simulink model "SCADA_Sawmill"  (R2024b)
settings: Solver=FixedStepAuto  StartTime=0.0  StopTime=Tsim  FixedStep=dT  RelTol=1e-3
values from neighbouring files (symbols this model uses):
  b = t + 2*s    (= 3.6)    [ParametriSegheria.m]    (also in ParametriSegheriaDinamica.m; main_param_CLASSIC.m; main_param_SCADA.m)
  change_cost = 60    [ParametriSegheriaDinamica.m]    (also in main_param_CLASSIC.m = 50; main_param_SCADA.m = 50)
  dT = 0.025    [ParametriSegheriaDinamica.m]    (also in main_param_CLASSIC.m; main_param_SCADA.m)
  h_index = [70, 80, 90, 100]    [ParametriSegheria.m]    (also in ParametriSegheriaDinamica.m = [80, 90, 100]; main_param_CLASSIC.m = [80, 90, 100, 110]; main_param_SCADA.m = [80, 90, 100, 110])
  h_start_1 = 1    [main_param_CLASSIC.m]
  h_start_2 = 2    [main_param_CLASSIC.m]
  h_start_3 = 3    [main_param_CLASSIC.m]
  h_start_4 = 1    [main_param_CLASSIC.m]
  h_start_5 = 2    [main_param_CLASSIC.m]
  h_start_6 = 3    [main_param_CLASSIC.m]
  J1 = 8*1e6    (= 8000000)    [ParametriSegheriaDinamica.m]    (also in main_param_CLASSIC.m; main_param_SCADA.m)
  J2 = 0.9*1e6    (= 900000)    [ParametriSegheriaDinamica.m]    (also in main_param_CLASSIC.m; main_param_SCADA.m)
  kc = [0 35 40 50 55 90]    [ParametriSegheria.m]    (also in ParametriSegheriaDinamica.m = [0, 25, 30, 35, 50, 70]; main_param_CLASSIC.m = [0, 25, 30, 35, 50, 70]; main_param_SCADA.m = [0, 25, 30, 35, 50, 70])
  Kt = 2    [ParametriSegheria.m]    (also in ParametriSegheriaDinamica.m = 10000; main_param_CLASSIC.m = 10000; main_param_SCADA.m = 10000)
  Kt2 = 5    [ParametriSegheria.m]    (also in ParametriSegheriaDinamica.m = 4500; main_param_CLASSIC.m = 4500; main_param_SCADA.m = 4500)
  l_index = [20, 30, 40, 50]    [ParametriSegheria.m]    (also in ParametriSegheriaDinamica.m = [30, 40, 50]; main_param_CLASSIC.m = [30, 40, 50, 60]; main_param_SCADA.m = [30, 40, 50, 60])
  l_start_1 = 1    [main_param_CLASSIC.m]
  l_start_2 = 1    [main_param_CLASSIC.m]
  l_start_3 = 1    [main_param_CLASSIC.m]
  l_start_4 = 1    [main_param_CLASSIC.m]
  l_start_5 = 1    [main_param_CLASSIC.m]
  l_start_6 = 1    [main_param_CLASSIC.m]
  Lt = 4    [ParametriSegheria.m]    (also in ParametriSegheriaDinamica.m; main_param_CLASSIC.m; main_param_SCADA.m)
  Mag_D1 = [0 randi([220 500], 1, 40)]    [ParametriSegheria.m]    (also in ParametriSegheriaDinamica.m = [0 randi([200 500], 1, N_log)]; main_param_CLASSIC.m = [0 randi([200 500], 1, N_log)]; main_param_SCADA.m = [0 randi([200 500], 1, N_log)])
  Mag_D2 = [0 randi([220 500], 1, 40)]    [ParametriSegheria.m]    (also in ParametriSegheriaDinamica.m = [0 randi([200 500], 1, N_log)]; main_param_CLASSIC.m = [0 randi([200 500], 1, N_log)]; main_param_SCADA.m = [0 randi([200 500], 1, N_log)])
  Mag_D3 = [0 randi([220 500], 1, 40)]    [ParametriSegheria.m]    (also in ParametriSegheriaDinamica.m = [0 randi([200 500], 1, N_log)]; main_param_CLASSIC.m = [0 randi([200 500], 1, N_log)]; main_param_SCADA.m = [0 randi([200 500], 1, N_log)])
  Mag_legno1 = [0 randi([1 5], 1, 40)]    [ParametriSegheria.m]    (also in ParametriSegheriaDinamica.m = [0 randi([1 5], 1, N_log)]; main_param_CLASSIC.m = [0 randi([1 5], 1, N_log)]; main_param_SCADA.m = [0 randi([1 5], 1, N_log)])
  Mag_legno2 = [0 randi([1 5], 1, 40)]    [ParametriSegheria.m]    (also in ParametriSegheriaDinamica.m = [0 randi([1 5], 1, N_log)]; main_param_CLASSIC.m = [0 randi([1 5], 1, N_log)]; main_param_SCADA.m = [0 randi([1 5], 1, N_log)])
  Mag_legno3 = [0 randi([1 5], 1, 40)]    [ParametriSegheria.m]    (also in ParametriSegheriaDinamica.m = [0 randi([1 5], 1, N_log)]; main_param_CLASSIC.m = [0 randi([1 5], 1, N_log)]; main_param_SCADA.m = [0 randi([1 5], 1, N_log)])
  n_linee = 3    [ParametriSegheriaDinamica.m]    (also in main_param_CLASSIC.m; main_param_SCADA.m)
  omega_ref1 = 50    [ParametriSegheriaDinamica.m]    (also in main_param_CLASSIC.m; main_param_SCADA.m)
  omega_ref2 = 3000*(2*pi/60)    (= 314.159265359)    [ParametriSegheriaDinamica.m]    (also in main_param_CLASSIC.m; main_param_SCADA.m)
  Rc = 200    [ParametriSegheria.m]    (also in ParametriSegheriaDinamica.m; main_param_CLASSIC.m; main_param_SCADA.m)
  rho = [0, 450, 520, 590, 710, 780]*1e-9    [ParametriSegheriaDinamica.m]    (also in main_param_CLASSIC.m; main_param_SCADA.m)
  Rs = 800    [ParametriSegheria.m]    (also in ParametriSegheriaDinamica.m; main_param_CLASSIC.m; main_param_SCADA.m)
  sigma_D = 10    [ParametriSegheriaDinamica.m]    (also in main_param_CLASSIC.m = 5; main_param_SCADA.m = 5)
  sigma_larg = 10    [ParametriSegheriaDinamica.m]    (also in main_param_CLASSIC.m = 5; main_param_SCADA.m = 5)
  SR = Rs/Rm    (= 5.33333333333)    [ParametriSegheria.m]    (also in ParametriSegheriaDinamica.m; main_param_CLASSIC.m; main_param_SCADA.m)
  SR2 = Rc/Rm2    (= 4)    [ParametriSegheria.m]    (also in ParametriSegheriaDinamica.m; main_param_CLASSIC.m; main_param_SCADA.m)
  target_matrice = randi([20, 120], length(h_index), length(l_index))    [ParametriSegheria.m]    (also in ParametriSegheriaDinamica.m = randi([20, 100], length(h_index), length(l_index)); main_param_CLASSIC.m = randi([20, 100], length(h_index), length(l_index)); main_param_SCADA.m = randi([20, 100], length(h_index), length(l_index)))
  thr_lavoro = 600000    [ParametriSegheriaDinamica.m]    (also in main_param_CLASSIC.m; main_param_SCADA.m)
  V_mean1 = 0.75    [ParametriSegheriaDinamica.m]    (also in main_param_CLASSIC.m; main_param_SCADA.m)
  V_mean23 = 1    [ParametriSegheriaDinamica.m]    (also in main_param_CLASSIC.m; main_param_SCADA.m)
libraries: simulink x24, slpidlib x18
(part 1 of 5)
settings Model: Creator=samue  LastModifiedBy=eliasantuari
settings SolverCC: EnableFixedStepZeroCrossing=on

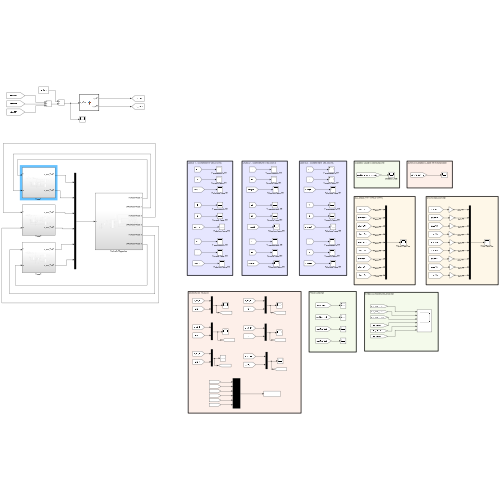
[thumbnail: Simulink's stored preview of the top-level diagram]
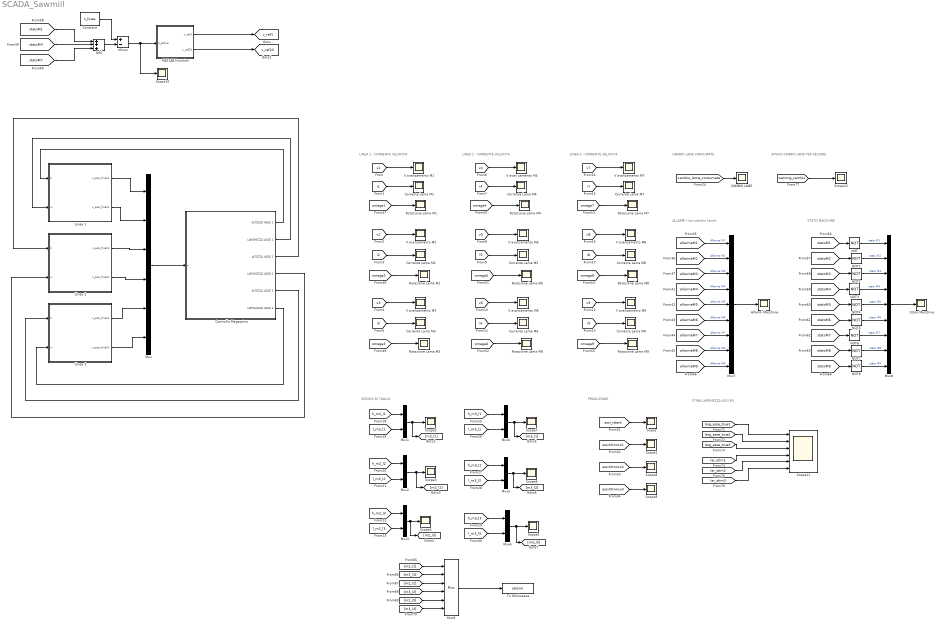
== system SCADA_Sawmill ==
  note: ALLARMI (non cambio lame)
  note: LINEA 2 - CORRENTE VELOCITA
  note: LINEA 1 - CORRENTE VELOCITA`
  note: LINEA 3 - CORRENTE VELOCITA
  note: SEZIONI DI TAGLIO
  note: CAMBIO LAME CONSUMATE
  note: PRODUZIONE
  note: STATO MACCHINE
  note: STIMA LARGHEZZA ASSI M1
  note: AVVISO CAMBIO LAME PER SEZIONE
  Add : Sum  Inputs=+++
  Allarmi Macchine : Scope
  CAMBIO LAME : Scope
  Constant : Constant  Value=n_linee
  Controllo Magazzino : Subsystem
  Corrente Lama M{1..9} (9 alike) : Scope
  Linea 1 : Subsystem
  Linea 2 : Subsystem
  Linea 3 : Subsystem
  MATLAB Function : MATLAB Function  TreatAsAtomicUnit=on
  Minus : Sum  Inputs=+-
  Mux : Mux  Inputs=6
  Mux{1..6} (6 alike) : Mux  Inputs=2
  Mux7 : Mux  Inputs=9
  Mux8 : Mux  Inputs=9
  Mux9 : Mux  Inputs=6
  NOT{,1..8} (9 alike) : Logic  Operator=NOT  IconShape=distinctive  AllPortsSameDT=off  OutDataTypeStr=boolean
  Rotazione Lama M{1..9} (9 alike) : Scope
  Scope{,1..10,12} (12 alike) : Scope
  Scope11 : Scope  NumInputPorts=6
  Stato Macchine : Scope
  To Workspace : ToWorkspace  VariableName=sezioni  SaveFormat=Timeseries  SampleTime=-1
  V avan zamento M4 : Scope
  V avanzamento M{1..3,5..9} (8 alike) : Scope
  tag scope: v_ref1=global, v_ref23=global
  wires:
  Linea 2/1(n_assi_finali1) -> Mux/3
  Controllo Magazzino/2(LARGHEZZA ASSE 1) -> Linea 1/2(w)
  Linea 2/2(n_assi_finali2) -> Mux/4
  [i9] -> Corrente Lama M9/1
  [v9] -> V avanzamento M9/1
  [i8] -> Corrente Lama M8/1
  [v7] -> V avanzamento M7/1
  [v8] -> V avanzamento M8/1
  [i7] -> Corrente Lama M7/1
  Controllo Magazzino/6(LARGHEZZA ASSE 3) -> Linea 3/2(w)
  Controllo Magazzino/3(ALTEZZA ASSE 2) -> Linea 2/1(h)
  [i3] -> Corrente Lama M3/1
  [v2] -> V avanzamento M2/1
  [v1] -> V avanzamento M1/1
  Controllo Magazzino/1(ALTEZZA ASSE 1) -> Linea 1/1(h)
  [i2] -> Corrente Lama M2/1
  [i1] -> Corrente Lama M1/1
  Linea 1/1(n_assi_finali1) -> Mux/1
  [v3] -> V avanzamento M3/1
  Mux/1 -> Controllo Magazzino/1(u)
  Linea 3/2(n_assi_finali2) -> Mux/6
  [i5] -> Corrente Lama M5/1
  [v5] -> V avanzamento M5/1
  Linea 3/1(n_assi_finali1) -> Mux/5
  Linea 1/2(n_assi_finali2) -> Mux/2
  [i4] -> Corrente Lama M4/1
  [v4] -> V avan zamento M4/1
  [v6] -> V avanzamento M6/1
  [i6] -> Corrente Lama M6/1
  Controllo Magazzino/5(ALTEZZA ASSE 3) -> Linea 3/1(h)
  Controllo Magazzino/4(LARGHEZZA ASSE 2) -> Linea 2/2(w)
  [cambio_lame_consumate] -> CAMBIO LAME/1
  [l_m2_l1] -> Mux1/2
  [h_m2_l1] -> Mux1/1
  Mux1/1 -> Scope2/1, [m2_l1]
  [h_m2_l2] -> Mux2/1
  [l_m2_l2] -> Mux2/2
  Mux2/1 -> [m2_l2], Scope3/1
  Mux3/1 -> Scope4/1, [m2_l3]
  [h_m2_l3] -> Mux3/1
  [l_m2_l3] -> Mux3/2
  Mux4/1 -> [m3_l3], Scope5/1
  [h_m3_l3] -> Mux4/1
  [l_m3_l3] -> Mux4/2
  Mux5/1 -> Scope6/1, [m3_l2]
  [h_m3_l2] -> Mux5/1
  [l_m3_l2] -> Mux5/2
  Mux6/1 -> [m3_l1], Scope7/1
  [h_m3_l1] -> Mux6/1
  [l_m3_l1] -> Mux6/2
  [assi_istant] -> Scope/1
  [assiXtronco1] -> Scope1/1
  [assiXtronco2] -> Scope8/1
  [assiXtronco3] -> Scope9/1
  [allarmeM3] -> Mux7/3  "Allarme M3"
  [allarmeM2] -> Mux7/2  "Allarme M2"
  Mux7/1 -> Allarmi Macchine/1
  [allarmeM1] -> Mux7/1  "Allarme M1"
  [allarmeM4] -> Mux7/4  "Allarme M4"
  [allarmeM5] -> Mux7/5  "Allarme M5"
  [allarmeM6] -> Mux7/6  "Allarme M6"
  [allarmeM9] -> Mux7/9  "Allarme M8"
  [allarmeM8] -> Mux7/8  "Allarme M4"
  [allarmeM7] -> Mux7/7  "Allarme M7"
  [statoM4] -> Add/2
  [statoM1] -> Add/1
  [statoM7] -> Add/3
  Add/1 -> Minus/2
  Constant/1 -> Minus/1
  Minus/1 -> Scope10/1, MATLAB Function/1(n_attive)
  MATLAB Function/1(v_ref1) -> [v_ref1]
  MATLAB Function/2(v_ref23) -> [v_ref23]
  [omega1] -> Rotazione Lama M1/1
  [omega2] -> Rotazione Lama M2/1
  [omega3] -> Rotazione Lama M3/1
  [omega4] -> Rotazione Lama M4/1
  [omega5] -> Rotazione Lama M5/1
  [omega6] -> Rotazione Lama M6/1
  [omega7] -> Rotazione Lama M7/1
  [omega8] -> Rotazione Lama M8/1
  [omega9] -> Rotazione Lama M9/1
  Mux8/1 -> Stato Macchine/1
  [statoM1] -> NOT/1
  NOT/1 -> Mux8/1  "stato M1"
  [statoM2] -> NOT1/1
  [statoM3] -> NOT2/1
  NOT1/1 -> Mux8/2  "stato M2"
  NOT2/1 -> Mux8/3  "stato M3"
  NOT5/1 -> Mux8/6  "stato M6"
  NOT4/1 -> Mux8/5  "stato M5"
  [statoM6] -> NOT5/1
  [statoM5] -> NOT4/1
  NOT3/1 -> Mux8/4  "stato M4"
  [statoM4] -> NOT3/1
  [statoM7] -> NOT6/1
  NOT6/1 -> Mux8/7  "stato M7"
  [statoM8] -> NOT7/1
  [statoM9] -> NOT8/1
  NOT7/1 -> Mux8/8  "stato M8"
  NOT8/1 -> Mux8/9  "stato M9"
  [m3_l1] -> Mux9/2
  Mux9/1 -> To Workspace/1
  [m2_l3] -> Mux9/5
  [m2_l2] -> Mux9/3
  [m3_l2] -> Mux9/4
  [m3_l3] -> Mux9/6
  [m2_l1] -> Mux9/1
  [larg_asse_true1] -> Scope11/1
  [larg_asse_true2] -> Scope11/2
  [larg_asse_true3] -> Scope11/3
  [lar_stim1] -> Scope11/4
  [lar_stim2] -> Scope11/5
  [lar_stim3] -> Scope11/6
  [warning_cambio] -> Scope12/1

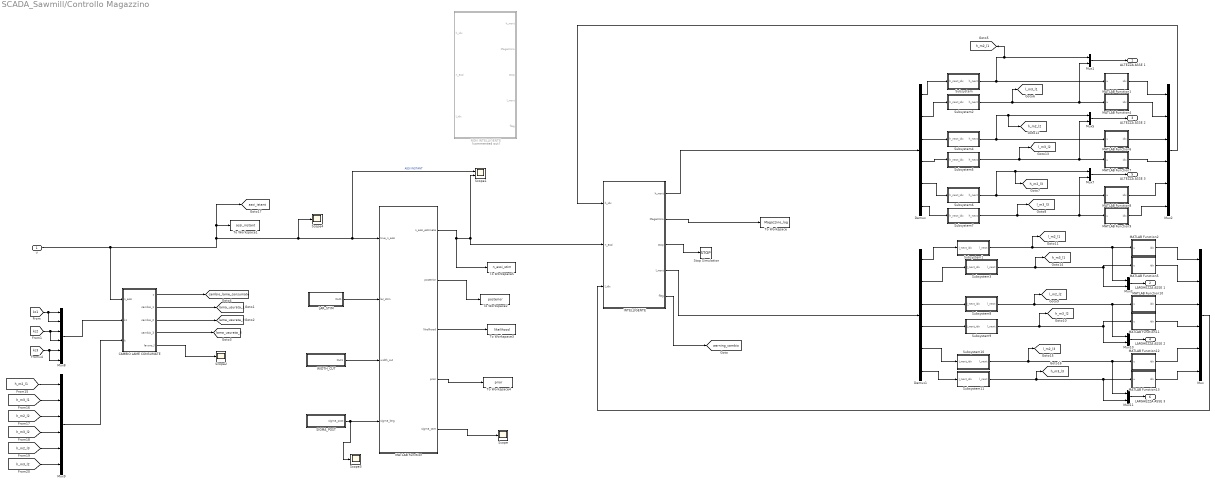
== system SCADA_Sawmill/Controllo Magazzino ==
  u : Inport
  CAMBIO LAME CONSUMATE : MATLAB Function  TreatAsAtomicUnit=on
  Demux : Demux  Outputs=6
  Demux1 : Demux  Outputs=6
  INTELLIGENTE : MATLAB Function  TreatAsAtomicUnit=on
  LAR_STIM : Subsystem
  MATLAB Function : MATLAB Function  TreatAsAtomicUnit=on
  MATLAB Function1 : MATLAB Function  TreatAsAtomicUnit=on
  MATLAB Function10 : MATLAB Function  TreatAsAtomicUnit=on
  MATLAB Function11 : MATLAB Function  TreatAsAtomicUnit=on
  MATLAB Function12 : MATLAB Function  TreatAsAtomicUnit=on
  MATLAB Function13 : MATLAB Function  TreatAsAtomicUnit=on
  MATLAB Function2 : MATLAB Function  TreatAsAtomicUnit=on
  MATLAB Function4 : MATLAB Function  TreatAsAtomicUnit=on
  MATLAB Function5 : MATLAB Function  TreatAsAtomicUnit=on
  MATLAB Function6 : MATLAB Function  TreatAsAtomicUnit=on
  MATLAB Function7 : MATLAB Function  TreatAsAtomicUnit=on
  MATLAB Function8 : MATLAB Function  TreatAsAtomicUnit=on
  MATLAB Function9 : MATLAB Function  TreatAsAtomicUnit=on
  Mux{,2,8..9} (4 alike) : Mux  Inputs=6
  Mux{1,3,5,7,10..11} (6 alike) : Mux  Inputs=2
  NON INTELLIGENTE : MATLAB Function  Commented=on  TreatAsAtomicUnit=on
  SIGMA_POST : Subsystem
  Scope{,2..4} (4 alike) : Scope
  Scope1 : Scope  NumInputPorts=2
  Stop Simulation : Stop
  Subsystem : Subsystem
  Subsystem1 : Subsystem
  Subsystem10 : Subsystem
  Subsystem11 : Subsystem
  Subsystem2 : Subsystem
  Subsystem3 : Subsystem
  Subsystem4 : Subsystem
  Subsystem5 : Subsystem
  Subsystem6 : Subsystem
  Subsystem7 : Subsystem
  Subsystem8 : Subsystem
  Subsystem9 : Subsystem
  To Workspace : ToWorkspace  VariableName=Magazzino_log  SaveFormat=Timeseries  SampleTime=-1
  To Workspace1 : ToWorkspace  VariableName=assi_instant  SaveFormat=Timeseries  SampleTime=-1
  To Workspace2 : ToWorkspace  VariableName=posterior  SaveFormat=Timeseries  SampleTime=-1
  To Workspace3 : ToWorkspace  VariableName=likelihood  SaveFormat=Timeseries  SampleTime=-1
  To Workspace4 : ToWorkspace  VariableName=prior  SaveFormat=Timeseries  SampleTime=-1
  To Workspace5 : ToWorkspace  VariableName=n_assi_stim  SaveFormat=Timeseries  SampleTime=-1
  WIDTH_CUT : Subsystem
  ALTEZZA ASSE 1 : Outport
  LARGHEZZA ASSE 1 : Outport  Port=2
  ALTEZZA ASSE 2 : Outport  Port=3
  LARGHEZZA ASSE 2 : Outport  Port=4
  ALTEZZA ASSE 3 : Outport  Port=5
  LARGHEZZA ASSE 3 : Outport  Port=6
  tag scope: assi_istant=global, cambio_lame_consumate=global, h_m2_l1=global, h_m2_l2=global, h_m2_l3=global, h_m3_l1=global, h_m3_l2=global, h_m3_l3=global, l_m2_l1=global, l_m2_l2=global, l_m2_l3=global, l_m3_l1=global, l_m3_l2=global, l_m3_l3=global, lama_usurata_1=global, lama_usurata_2=global, lama_usurata_3=global, warning_cambio=global
  wires:
  Subsystem/1(h_next) -> Mux1/1, [h_m2_l1], MATLAB Function1/1(u)
  Subsystem1/1(l_next) -> [l_m2_l1], Mux3/1, MATLAB Function2/1(u)
  Subsystem2/1(h_next) -> Mux1/2, MATLAB Function4/1(u), [l_m3_l1]
  Demux/2 -> Subsystem2/1(h_next_idx)
  Demux/1 -> Subsystem/1(h_next_idx)
  Mux1/1 -> ALTEZZA ASSE 1/1
  Subsystem3/1(l_next) -> [h_m3_l1], MATLAB Function5/1(u), Mux3/2
  Mux3/1 -> LARGHEZZA ASSE 1/1
  Subsystem5/1(h_next) -> [l_m3_l2], Mux5/2, MATLAB Function7/1(u)
  Mux5/1 -> ALTEZZA ASSE 2/1
  Subsystem4/1(h_next) -> [h_m2_l2], Mux5/1, MATLAB Function6/1(u)
  Subsystem7/1(h_next) -> [l_m3_l3], Mux7/2, MATLAB Function9/1(u)
  Mux7/1 -> ALTEZZA ASSE 3/1
  Subsystem6/1(h_next) -> [h_m2_l3], Mux7/1, MATLAB Function8/1(u)
  Demux/3 -> Subsystem4/1(h_next_idx)
  Demux/4 -> Subsystem5/1(h_next_idx)
  Demux/5 -> Subsystem6/1(h_next_idx)
  Demux/6 -> Subsystem7/1(h_next_idx)
  Mux10/1 -> LARGHEZZA ASSE 2/1
  Subsystem9/1(l_next) -> [h_m3_l2], MATLAB Function11/1(u), Mux10/2
  Subsystem8/1(l_next) -> [l_m2_l2], MATLAB Function10/1(u), Mux10/1
  Subsystem10/1(l_next) -> [l_m2_l3], Mux11/1, MATLAB Function12/1(u)
  Subsystem11/1(l_next) -> [h_m3_l3], Mux11/2, MATLAB Function13/1(u)
  Mux11/1 -> LARGHEZZA ASSE 3/1
  Demux1/1 -> Subsystem1/1(I_next_idx)
  Demux1/2 -> Subsystem3/1(I_next_idx)
  Demux1/3 -> Subsystem8/1(I_next_idx)
  Demux1/4 -> Subsystem9/1(I_next_idx)
  Demux1/5 -> Subsystem10/1(I_next_idx)
  Demux1/6 -> Subsystem11/1(I_next_idx)
  MATLAB Function2/1(idx) -> Mux/1
  MATLAB Function5/1(idx) -> Mux/2
  MATLAB Function10/1(idx) -> Mux/3
  MATLAB Function11/1(idx) -> Mux/4
  MATLAB Function12/1(idx) -> Mux/5
  MATLAB Function13/1(idx) -> Mux/6
  Mux/1 -> INTELLIGENTE/3(l_idx)
  MATLAB Function1/1(idx) -> Mux2/1
  MATLAB Function4/1(idx) -> Mux2/2
  MATLAB Function6/1(idx) -> Mux2/3
  MATLAB Function7/1(idx) -> Mux2/4
  MATLAB Function8/1(idx) -> Mux2/5
  MATLAB Function9/1(idx) -> Mux2/6
  Mux2/1 -> INTELLIGENTE/1(h_idx)
  INTELLIGENTE/2(Magazzino) -> To Workspace/1
  INTELLIGENTE/1(h_next) -> Demux/1
  INTELLIGENTE/4(l_next) -> Demux1/1
  INTELLIGENTE/3(stop) -> Stop Simulation/1
  MATLAB Function/2(posterior) -> To Workspace2/1
  MATLAB Function/3(likelihood) -> To Workspace3/1
  MATLAB Function/4(prior) -> To Workspace4/1
  [h_m3_l2] -> Mux9/6
  CAMBIO LAME CONSUMATE/3(cambio_2) -> [lama_usurata_2]
  [kc3] -> Mux8/6, Mux8/5
  u/1 -> CAMBIO LAME CONSUMATE/1(n_assi), Scope4/1, Scope1/1, MATLAB Function/1(true_n_assi), To Workspace1/1, [assi_istant]  "ASSI INSTANT"
  [kc1] -> Mux8/2, Mux8/1
  [kc2] -> Mux8/4, Mux8/3
  CAMBIO LAME CONSUMATE/4(cambio_3) -> [lama_usurata_3]
  CAMBIO LAME CONSUMATE/1(y) -> [cambio_lame_consumate]
  Mux8/1 -> CAMBIO LAME CONSUMATE/2(kc)
  [h_m2_l2] -> Mux9/3
  Mux9/1 -> CAMBIO LAME CONSUMATE/3(h)
  CAMBIO LAME CONSUMATE/5(lavoro_l) -> Scope2/1
  CAMBIO LAME CONSUMATE/2(cambio_1) -> [lama_usurata_1]
  [h_m3_l1] -> Mux9/2
  [h_m3_l2] -> Mux9/4
  [h_m2_l1] -> Mux9/1
  [h_m2_l3] -> Mux9/5
  WIDTH_CUT/1(Out1) -> MATLAB Function/3(width_cut)
  LAR_STIM/1(Out1) -> MATLAB Function/2(lar_stim)
  SIGMA_POST/1(sigma_post) -> Scope3/1, MATLAB Function/4(sigma_larg)
  MATLAB Function/1(n_assi_estimate) -> INTELLIGENTE/2(n_assi), Scope1/2, To Workspace5/1
  INTELLIGENTE/5(flag) -> [warning_cambio]
  MATLAB Function/5(sigma_cam) -> Scope/1

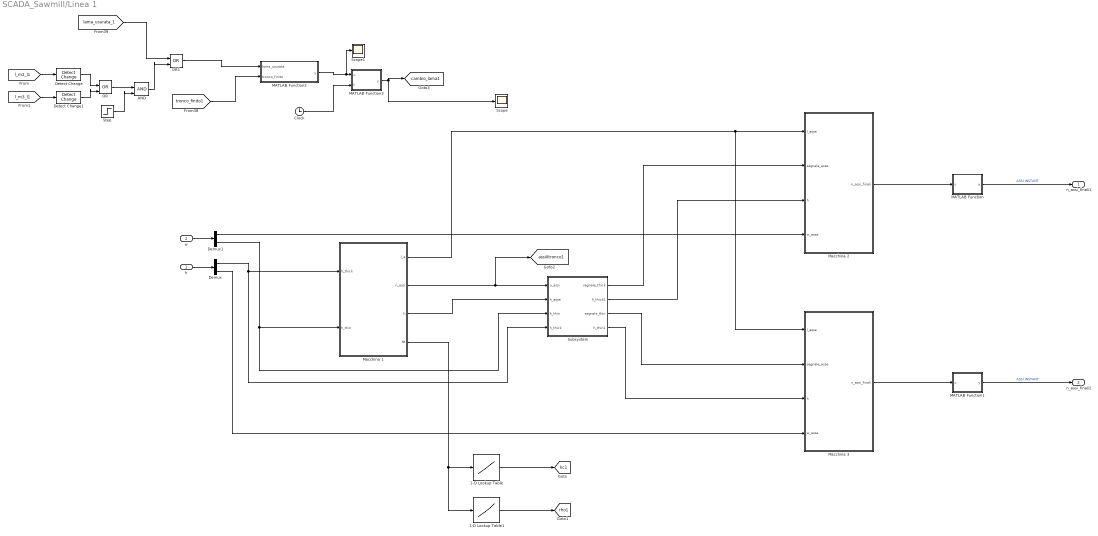
== system SCADA_Sawmill/Linea 1 ==
  h : Inport
  w : Inport  Port=2
  1-D Lookup Table : Lookup_n-D  NumberOfTableDimensions=1  BreakpointsForDimension1=[0 1 2 3 4 5 ]  Table=kc  InternalRulePriority=Speed  RndMeth=Simplest
  1-D Lookup Table1 : Lookup_n-D  NumberOfTableDimensions=1  BreakpointsForDimension1=[0 1 2 3 4 5 ]  Table=rho  InternalRulePriority=Speed  RndMeth=Simplest
  AND : Logic  IconShape=distinctive  AllPortsSameDT=off  OutDataTypeStr=boolean
  Clock : Clock
  Demux : Demux  Outputs=2
  Demux1 : Demux  Outputs=2
  Detect Change : simulink/Logic and Bit Operations/Detect Change  vinit=0  OutDataTypeStr=boolean
  Detect Change1 : simulink/Logic and Bit Operations/Detect Change  vinit=0  OutDataTypeStr=boolean
  MATLAB Function : MATLAB Function  TreatAsAtomicUnit=on
  MATLAB Function1 : MATLAB Function  TreatAsAtomicUnit=on
  MATLAB Function2 : MATLAB Function  TreatAsAtomicUnit=on
  MATLAB Function3 : MATLAB Function  TreatAsAtomicUnit=on
  Macchina 1 : Subsystem
  Macchina 2 : Subsystem
  Macchina 3 : Subsystem
  OR : Logic  Operator=OR  IconShape=distinctive  AllPortsSameDT=off  OutDataTypeStr=boolean
  OR1 : Logic  Operator=OR  IconShape=distinctive  AllPortsSameDT=off  OutDataTypeStr=boolean
  Scope : Scope
  Scope1 : Scope
  Step : Step  Time=2*dT  SampleTime=0
  Subsystem : Subsystem
  n_assi_finali1 : Outport
  n_assi_finali2 : Outport  Port=2
  tag scope: assiXtronco1=global, cambio_lama1=global, kc1=global, rho1=global
  wires:
  Macchina 1/1(l_a) -> Macchina 3/1(l_asse), Macchina 2/1(l_asse)
  Macchina 1/2(n_assi) -> [assiXtronco1], Subsystem/1(n_assi)
  Macchina 1/3(h) -> Subsystem/2(h_asse)
  Macchina 3/1(n_assi_finali) -> MATLAB Function1/1(u)
  Macchina 2/1(n_assi_finali) -> MATLAB Function/1(u)
  MATLAB Function/1(y) -> n_assi_finali1/1  "ASSI INSTANT"
  MATLAB Function1/1(y) -> n_assi_finali2/1  "ASSI INSTANT"
  Subsystem/1(segnale_thick) -> Macchina 2/2(segnale_asse)
  Subsystem/2(h_thick1) -> Macchina 2/3(h)
  Subsystem/3(segnale_thin) -> Macchina 3/2(segnale_asse)
  Subsystem/4(h_thin1) -> Macchina 3/3(h)
  1-D Lookup Table/1 -> [kc1]
  1-D Lookup Table1/1 -> [rho1]
  Macchina 1/4(Nt) -> 1-D Lookup Table1/1, 1-D Lookup Table/1
  h/1 -> Demux/1
  w/1 -> Demux1/1
  Demux/2 -> Macchina 3/4(w_asse)
  Demux/1 -> Macchina 1/1(h_thick), Subsystem/4(h_thick)
  Demux1/1 -> Macchina 2/4(w_asse)
  Demux1/2 -> Subsystem/3(h_thin), Macchina 1/2(h_thin)
  MATLAB Function3/1(y) -> [cambio_lama1], Scope/1
  [tronco_finito1] -> MATLAB Function2/2(tronco_finito)
  Clock/1 -> MATLAB Function3/2(t)
  MATLAB Function2/1(y) -> Scope1/1, MATLAB Function3/1(u)
  [lama_usurata_1] -> OR1/1
  Detect Change/1 -> OR/1
  OR/1 -> AND/1
  Step/1 -> AND/2
  Detect Change1/1 -> OR/2
  AND/1 -> OR1/2
  [l_m3_l1] -> Detect Change1/1
  [l_m2_l1] -> Detect Change/1
  OR1/1 -> MATLAB Function2/1(lama_usurata)

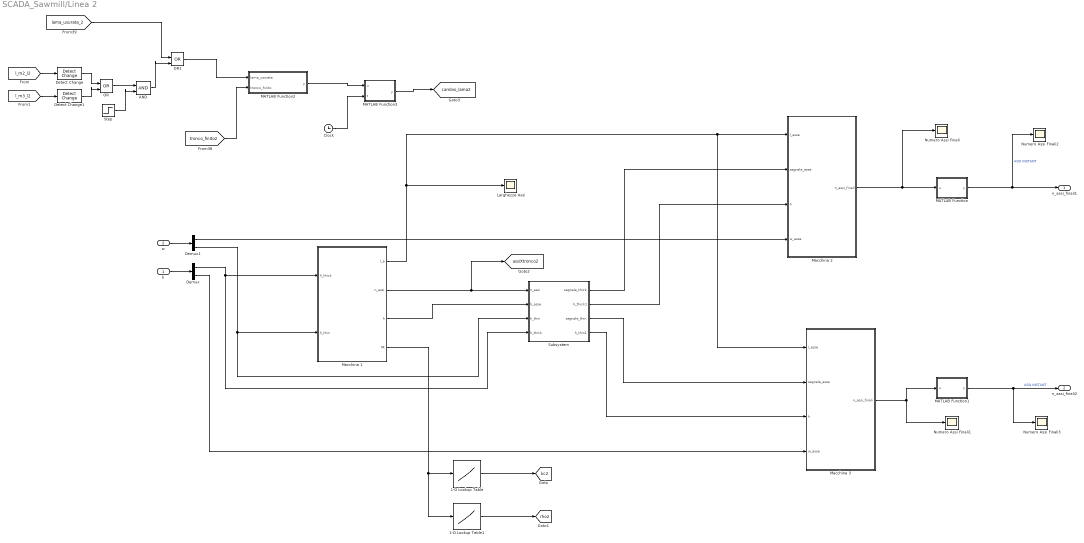
== system SCADA_Sawmill/Linea 2 ==
  h : Inport
  w : Inport  Port=2
  1-D Lookup Table : Lookup_n-D  NumberOfTableDimensions=1  BreakpointsForDimension1=[0 1 2 3 4 5 ]  Table=kc  InternalRulePriority=Speed  RndMeth=Simplest
  1-D Lookup Table1 : Lookup_n-D  NumberOfTableDimensions=1  BreakpointsForDimension1=[0 1 2 3 4 5 ]  Table=rho  InternalRulePriority=Speed  RndMeth=Simplest
  AND : Logic  IconShape=distinctive  AllPortsSameDT=off  OutDataTypeStr=boolean
  Clock : Clock
  Demux : Demux  Outputs=2
  Demux1 : Demux  Outputs=2
  Detect Change : simulink/Logic and Bit Operations/Detect Change  vinit=0  OutDataTypeStr=boolean
  Detect Change1 : simulink/Logic and Bit Operations/Detect Change  vinit=0  OutDataTypeStr=boolean
  Larghezze Assi : Scope
  MATLAB Function : MATLAB Function  TreatAsAtomicUnit=on
  MATLAB Function1 : MATLAB Function  TreatAsAtomicUnit=on
  MATLAB Function2 : MATLAB Function  TreatAsAtomicUnit=on
  MATLAB Function3 : MATLAB Function  TreatAsAtomicUnit=on
  Macchina 1 : Subsystem
  Macchina 2 : Subsystem
  Macchina 3 : Subsystem
  Numero Assi Finali{,1..3} (4 alike) : Scope
  OR : Logic  Operator=OR  IconShape=distinctive  AllPortsSameDT=off  OutDataTypeStr=boolean
  OR1 : Logic  Operator=OR  IconShape=distinctive  AllPortsSameDT=off  OutDataTypeStr=boolean
  Step : Step  Time=2*dT  SampleTime=0
  Subsystem : Subsystem
  n_assi_finali1 : Outport
  n_assi_finali2 : Outport  Port=2
  tag scope: assiXtronco2=global, cambio_lama2=global, kc2=global, rho2=global
  wires:
  Demux1/2 -> Macchina 1/2(h_thin), Subsystem/3(h_thin)
  Demux1/1 -> Macchina 2/4(w_asse)
  Demux/1 -> Subsystem/4(h_thick), Macchina 1/1(h_thick)
  Demux/2 -> Macchina 3/4(w_asse)
  w/1 -> Demux1/1
  h/1 -> Demux/1
  Macchina 1/4(Nt) -> 1-D Lookup Table/1, 1-D Lookup Table1/1
  1-D Lookup Table1/1 -> [rho2]
  1-D Lookup Table/1 -> [kc2]
  Subsystem/4(h_thin1) -> Macchina 3/3(h)
  Subsystem/3(segnale_thin) -> Macchina 3/2(segnale_asse)
  Subsystem/2(h_thick1) -> Macchina 2/3(h)
  Subsystem/1(segnale_thick) -> Macchina 2/2(segnale_asse)
  MATLAB Function1/1(y) -> n_assi_finali2/1, Numero Assi Finali3/1  "ASSI INSTANT"
  MATLAB Function/1(y) -> n_assi_finali1/1, Numero Assi Finali2/1  "ASSI INSTANT"
  Macchina 2/1(n_assi_finali) -> MATLAB Function/1(u), Numero Assi Finali/1
  Macchina 3/1(n_assi_finali) -> MATLAB Function1/1(u), Numero Assi Finali1/1
  Macchina 1/3(h) -> Subsystem/2(h_asse)
  Macchina 1/2(n_assi) -> [assiXtronco2], Subsystem/1(n_assi)
  Macchina 1/1(l_a) -> Macchina 2/1(l_asse), Macchina 3/1(l_asse), Larghezze Assi/1
  [tronco_finito2] -> MATLAB Function2/2(tronco_finito)
  Clock/1 -> MATLAB Function3/2(t)
  MATLAB Function2/1(y) -> MATLAB Function3/1(u)
  MATLAB Function3/1(y) -> [cambio_lama2]
  [l_m2_l2] -> Detect Change/1
  [l_m3_l2] -> Detect Change1/1
  Detect Change/1 -> OR/1
  Detect Change1/1 -> OR/2
  OR/1 -> AND/1
  Step/1 -> AND/2
  [lama_usurata_2] -> OR1/1
  AND/1 -> OR1/2
  OR1/1 -> MATLAB Function2/1(lama_usurata)

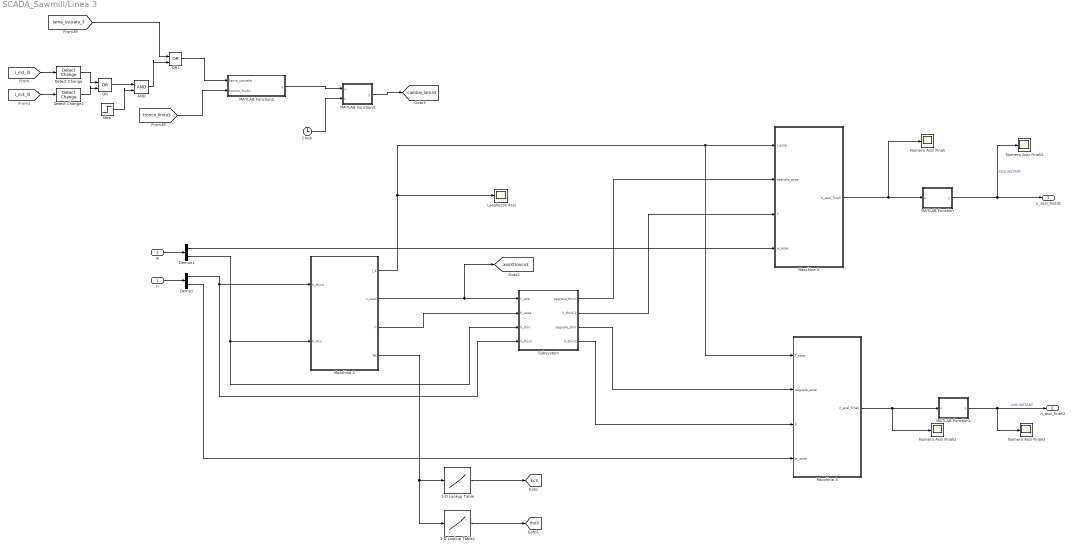
== system SCADA_Sawmill/Linea 3 ==
  h : Inport
  w : Inport  Port=2
  1-D Lookup Table : Lookup_n-D  NumberOfTableDimensions=1  BreakpointsForDimension1=[0 1 2 3 4 5 ]  Table=kc  InternalRulePriority=Speed  RndMeth=Simplest
  1-D Lookup Table1 : Lookup_n-D  NumberOfTableDimensions=1  BreakpointsForDimension1=[0 1 2 3 4 5 ]  Table=rho  InternalRulePriority=Speed  RndMeth=Simplest
  AND : Logic  IconShape=distinctive  AllPortsSameDT=off  OutDataTypeStr=boolean
  Clock : Clock
  Demux : Demux  Outputs=2
  Demux1 : Demux  Outputs=2
  Detect Change : simulink/Logic and Bit Operations/Detect Change  vinit=0  OutDataTypeStr=boolean
  Detect Change1 : simulink/Logic and Bit Operations/Detect Change  vinit=0  OutDataTypeStr=boolean
  Larghezze Assi : Scope
  MATLAB Function : MATLAB Function  TreatAsAtomicUnit=on
  MATLAB Function1 : MATLAB Function  TreatAsAtomicUnit=on
  MATLAB Function2 : MATLAB Function  TreatAsAtomicUnit=on
  MATLAB Function3 : MATLAB Function  TreatAsAtomicUnit=on
  Macchina 1 : Subsystem
  Macchina 2 : Subsystem
  Macchina 3 : Subsystem
  Numero Assi Finali{,1..3} (4 alike) : Scope
  OR : Logic  Operator=OR  IconShape=distinctive  AllPortsSameDT=off  OutDataTypeStr=boolean
  OR1 : Logic  Operator=OR  IconShape=distinctive  AllPortsSameDT=off  OutDataTypeStr=boolean
  Step : Step  Time=2*dT  SampleTime=0
  Subsystem : Subsystem
  n_assi_finali1 : Outport
  n_assi_finali2 : Outport  Port=2
  tag scope: assiXtronco3=global, cambio_lama3=global, kc3=global, rho3=global
  wires:
  Macchina 1/1(l_a) -> Larghezze Assi/1, Macchina 3/1(l_asse), Macchina 2/1(l_asse)
  Macchina 1/2(n_assi) -> [assiXtronco3], Subsystem/1(n_assi)
  Macchina 1/3(h) -> Subsystem/2(h_asse)
  Macchina 3/1(n_assi_finali) -> Numero Assi Finali1/1, MATLAB Function1/1(u)
  Macchina 2/1(n_assi_finali) -> Numero Assi Finali/1, MATLAB Function/1(u)
  MATLAB Function/1(y) -> Numero Assi Finali2/1, n_assi_finali1/1  "ASSI INSTANT"
  MATLAB Function1/1(y) -> n_assi_finali2/1, Numero Assi Finali3/1  "ASSI INSTANT"
  Subsystem/1(segnale_thick) -> Macchina 2/2(segnale_asse)
  Subsystem/2(h_thick1) -> Macchina 2/3(h)
  Subsystem/3(segnale_thin) -> Macchina 3/2(segnale_asse)
  Subsystem/4(h_thin1) -> Macchina 3/3(h)
  1-D Lookup Table/1 -> [kc3]
  1-D Lookup Table1/1 -> [rho3]
  Macchina 1/4(Nt) -> 1-D Lookup Table1/1, 1-D Lookup Table/1
  h/1 -> Demux/1
  w/1 -> Demux1/1
  Demux/2 -> Macchina 3/4(w_asse)
  Demux/1 -> Macchina 1/1(h_thick), Subsystem/4(h_thick)
  Demux1/1 -> Macchina 2/4(w_asse)
  Demux1/2 -> Subsystem/3(h_thin), Macchina 1/2(h_thin)
  [tronco_finito3] -> MATLAB Function2/2(tronco_finito)
  MATLAB Function2/1(y) -> MATLAB Function3/1(u)
  Clock/1 -> MATLAB Function3/2(t)
  MATLAB Function3/1(y) -> [cambio_lama3]
  [lama_usurata_3] -> OR1/1
  Detect Change/1 -> OR/1
  OR/1 -> AND/1
  Step/1 -> AND/2
  Detect Change1/1 -> OR/2
  AND/1 -> OR1/2
  [l_m3_l3] -> Detect Change1/1
  [l_m2_l3] -> Detect Change/1
  OR1/1 -> MATLAB Function2/1(lama_usurata)

== system SCADA_Sawmill/Controllo Magazzino/LAR_STIM ==
  Mux4 : Mux  Inputs=6
  Out1 : Outport
  wires:
  [lar_stim2] -> Mux4/3
  [lar_stim1] -> Mux4/1
  [lar_stim2] -> Mux4/4
  [lar_stim3] -> Mux4/6
  [lar_stim1] -> Mux4/2
  Mux4/1 -> Out1/1
  [lar_stim3] -> Mux4/5

== system SCADA_Sawmill/Controllo Magazzino/SIGMA_POST ==
  Mux6 : Mux  Inputs=6
  sigma_post : Outport
  wires:
  Mux6/1 -> sigma_post/1
  [sigma_post2] -> Mux6/3
  [sigma_post3] -> Mux6/5
  [sigma_post1] -> Mux6/1
  [sigma_post2] -> Mux6/4
  [sigma_post1] -> Mux6/2
  [sigma_post3] -> Mux6/6

== system SCADA_Sawmill/Controllo Magazzino/Subsystem ==
  h_next_idx : Inport
  Constant4 : Constant  Value=h_index
  Constant7 : Constant  Value=h_start_1
  Memory : Memory
  SELEZIONE ALTEZZA : Selector  InputPortWidth=length(h_index)  IndexOptions=Index vector (port)  Indices=[1 3]  OutputSizes=1
  Switch1 : Switch  Criteria=u2 > Threshold  SaturateOnIntegerOverflow=off  InputSameDT=off
  h_next : Outport
  wires:
  h_next_idx/1 -> Memory/1
  Constant7/1 -> Switch1/3
  Memory/1 -> Switch1/2, Switch1/1
  SELEZIONE ALTEZZA/1 -> h_next/1
  Constant4/1 -> SELEZIONE ALTEZZA/1
  Switch1/1 -> SELEZIONE ALTEZZA/2

== system SCADA_Sawmill/Controllo Magazzino/Subsystem1 ==
  I_next_idx : Inport
  Constant5 : Constant  Value=l_index
  Constant8 : Constant  Value=l_start_1
  Memory1 : Memory
  SELEZIONE LUNGHEZZA : Selector  InputPortWidth=length(h_index)  IndexOptions=Index vector (port)  Indices=[1 3]  OutputSizes=1
  Switch2 : Switch  Criteria=u2 > Threshold  SaturateOnIntegerOverflow=off  InputSameDT=off
  l_next : Outport
  wires:
  Memory1/1 -> Switch2/1, Switch2/2
  SELEZIONE LUNGHEZZA/1 -> l_next/1
  Switch2/1 -> SELEZIONE LUNGHEZZA/2
  Constant5/1 -> SELEZIONE LUNGHEZZA/1
  I_next_idx/1 -> Memory1/1
  Constant8/1 -> Switch2/3

== system SCADA_Sawmill/Controllo Magazzino/Subsystem10 ==
  I_next_idx : Inport
  Constant5 : Constant  Value=l_index
  Constant8 : Constant  Value=l_start_3
  Memory1 : Memory
  SELEZIONE LUNGHEZZA : Selector  InputPortWidth=length(h_index)  IndexOptions=Index vector (port)  Indices=[1 3]  OutputSizes=1
  Switch2 : Switch  Criteria=u2 > Threshold  SaturateOnIntegerOverflow=off  InputSameDT=off
  l_next : Outport
  wires:
  Memory1/1 -> Switch2/1, Switch2/2
  SELEZIONE LUNGHEZZA/1 -> l_next/1
  Switch2/1 -> SELEZIONE LUNGHEZZA/2
  Constant5/1 -> SELEZIONE LUNGHEZZA/1
  I_next_idx/1 -> Memory1/1
  Constant8/1 -> Switch2/3

== system SCADA_Sawmill/Controllo Magazzino/Subsystem11 ==
  I_next_idx : Inport
  Constant5 : Constant  Value=l_index
  Constant8 : Constant  Value=l_start_6
  Memory1 : Memory
  SELEZIONE LUNGHEZZA : Selector  InputPortWidth=length(h_index)  IndexOptions=Index vector (port)  Indices=[1 3]  OutputSizes=1
  Switch2 : Switch  Criteria=u2 > Threshold  SaturateOnIntegerOverflow=off  InputSameDT=off
  l_next : Outport
  wires:
  Constant8/1 -> Switch2/3
  I_next_idx/1 -> Memory1/1
  Constant5/1 -> SELEZIONE LUNGHEZZA/1
  Switch2/1 -> SELEZIONE LUNGHEZZA/2
  SELEZIONE LUNGHEZZA/1 -> l_next/1
  Memory1/1 -> Switch2/2, Switch2/1

== system SCADA_Sawmill/Controllo Magazzino/Subsystem2 ==
  h_next_idx : Inport
  Constant4 : Constant  Value=h_index
  Constant7 : Constant  Value=h_start_4
  Memory : Memory
  SELEZIONE ALTEZZA : Selector  InputPortWidth=length(h_index)  IndexOptions=Index vector (port)  Indices=[1 3]  OutputSizes=1
  Switch1 : Switch  Criteria=u2 > Threshold  SaturateOnIntegerOverflow=off  InputSameDT=off
  h_next : Outport
  wires:
  Switch1/1 -> SELEZIONE ALTEZZA/2
  Constant4/1 -> SELEZIONE ALTEZZA/1
  SELEZIONE ALTEZZA/1 -> h_next/1
  Memory/1 -> Switch1/1, Switch1/2
  Constant7/1 -> Switch1/3
  h_next_idx/1 -> Memory/1

== system SCADA_Sawmill/Controllo Magazzino/Subsystem3 ==
  I_next_idx : Inport
  Constant1 : Constant  Value=l_start_4
  Constant5 : Constant  Value=l_index
  Memory1 : Memory
  SELEZIONE LUNGHEZZA : Selector  InputPortWidth=length(h_index)  IndexOptions=Index vector (port)  Indices=[1 3]  OutputSizes=1
  Switch2 : Switch  Criteria=u2 > Threshold  SaturateOnIntegerOverflow=off  InputSameDT=off
  l_next : Outport
  wires:
  Constant1/1 -> Switch2/3
  I_next_idx/1 -> Memory1/1
  Constant5/1 -> SELEZIONE LUNGHEZZA/1
  Switch2/1 -> SELEZIONE LUNGHEZZA/2
  SELEZIONE LUNGHEZZA/1 -> l_next/1
  Memory1/1 -> Switch2/2, Switch2/1

== system SCADA_Sawmill/Controllo Magazzino/Subsystem4 ==
  h_next_idx : Inport
  Constant4 : Constant  Value=h_index
  Constant7 : Constant  Value=h_start_2
  Memory : Memory
  SELEZIONE ALTEZZA : Selector  InputPortWidth=length(h_index)  IndexOptions=Index vector (port)  Indices=[1 3]  OutputSizes=1
  Switch1 : Switch  Criteria=u2 > Threshold  SaturateOnIntegerOverflow=off  InputSameDT=off
  h_next : Outport
  wires:
  h_next_idx/1 -> Memory/1
  Constant7/1 -> Switch1/3
  Memory/1 -> Switch1/2, Switch1/1
  SELEZIONE ALTEZZA/1 -> h_next/1
  Constant4/1 -> SELEZIONE ALTEZZA/1
  Switch1/1 -> SELEZIONE ALTEZZA/2

== system SCADA_Sawmill/Controllo Magazzino/Subsystem5 ==
  h_next_idx : Inport
  Constant4 : Constant  Value=h_index
  Constant7 : Constant  Value=h_start_5
  Memory : Memory
  SELEZIONE ALTEZZA : Selector  InputPortWidth=length(h_index)  IndexOptions=Index vector (port)  Indices=[1 3]  OutputSizes=1
  Switch1 : Switch  Criteria=u2 > Threshold  SaturateOnIntegerOverflow=off  InputSameDT=off
  h_next : Outport
  wires:
  Switch1/1 -> SELEZIONE ALTEZZA/2
  Constant4/1 -> SELEZIONE ALTEZZA/1
  SELEZIONE ALTEZZA/1 -> h_next/1
  Memory/1 -> Switch1/1, Switch1/2
  Constant7/1 -> Switch1/3
  h_next_idx/1 -> Memory/1

== system SCADA_Sawmill/Controllo Magazzino/Subsystem6 ==
  h_next_idx : Inport
  Constant4 : Constant  Value=h_index
  Constant7 : Constant  Value=h_start_3
  Memory : Memory
  SELEZIONE ALTEZZA : Selector  InputPortWidth=length(h_index)  IndexOptions=Index vector (port)  Indices=[1 3]  OutputSizes=1
  Switch1 : Switch  Criteria=u2 > Threshold  SaturateOnIntegerOverflow=off  InputSameDT=off
  h_next : Outport
  wires:
  h_next_idx/1 -> Memory/1
  Constant7/1 -> Switch1/3
  Memory/1 -> Switch1/2, Switch1/1
  SELEZIONE ALTEZZA/1 -> h_next/1
  Constant4/1 -> SELEZIONE ALTEZZA/1
  Switch1/1 -> SELEZIONE ALTEZZA/2

== system SCADA_Sawmill/Controllo Magazzino/Subsystem7 ==
  h_next_idx : Inport
  Constant4 : Constant  Value=h_index
  Constant7 : Constant  Value=h_start_6
  Memory : Memory
  SELEZIONE ALTEZZA : Selector  InputPortWidth=length(h_index)  IndexOptions=Index vector (port)  Indices=[1 3]  OutputSizes=1
  Switch1 : Switch  Criteria=u2 > Threshold  SaturateOnIntegerOverflow=off  InputSameDT=off
  h_next : Outport
  wires:
  Switch1/1 -> SELEZIONE ALTEZZA/2
  Constant4/1 -> SELEZIONE ALTEZZA/1
  SELEZIONE ALTEZZA/1 -> h_next/1
  Memory/1 -> Switch1/1, Switch1/2
  Constant7/1 -> Switch1/3
  h_next_idx/1 -> Memory/1

== system SCADA_Sawmill/Controllo Magazzino/Subsystem8 ==
  I_next_idx : Inport
  Constant5 : Constant  Value=l_index
  Constant8 : Constant  Value=l_start_2
  Memory1 : Memory
  SELEZIONE LUNGHEZZA : Selector  InputPortWidth=length(h_index)  IndexOptions=Index vector (port)  Indices=[1 3]  OutputSizes=1
  Switch2 : Switch  Criteria=u2 > Threshold  SaturateOnIntegerOverflow=off  InputSameDT=off
  l_next : Outport
  wires:
  Constant8/1 -> Switch2/3
  I_next_idx/1 -> Memory1/1
  Constant5/1 -> SELEZIONE LUNGHEZZA/1
  Switch2/1 -> SELEZIONE LUNGHEZZA/2
  SELEZIONE LUNGHEZZA/1 -> l_next/1
  Memory1/1 -> Switch2/2, Switch2/1

== system SCADA_Sawmill/Controllo Magazzino/Subsystem9 ==
  I_next_idx : Inport
  Constant5 : Constant  Value=l_index
  Constant8 : Constant  Value=l_start_5
  Memory1 : Memory
  SELEZIONE LUNGHEZZA : Selector  InputPortWidth=length(h_index)  IndexOptions=Index vector (port)  Indices=[1 3]  OutputSizes=1
  Switch2 : Switch  Criteria=u2 > Threshold  SaturateOnIntegerOverflow=off  InputSameDT=off
  l_next : Outport
  wires:
  Memory1/1 -> Switch2/1, Switch2/2
  SELEZIONE LUNGHEZZA/1 -> l_next/1
  Switch2/1 -> SELEZIONE LUNGHEZZA/2
  Constant5/1 -> SELEZIONE LUNGHEZZA/1
  I_next_idx/1 -> Memory1/1
  Constant8/1 -> Switch2/3

== system SCADA_Sawmill/Controllo Magazzino/WIDTH_CUT ==
  Mux6 : Mux  Inputs=6
  Out1 : Outport
  wires:
  Mux6/1 -> Out1/1
  [w_cut_m2_l2] -> Mux6/3
  [w_cut_m2_l3] -> Mux6/5
  [w_cut_m2_l1] -> Mux6/1
  [w_cut_m3_l2] -> Mux6/4
  [w_cut_m3_l1] -> Mux6/2
  [w_cut_m3_l3] -> Mux6/6

== system SCADA_Sawmill/Linea 1/Macchina 1 ==
  h_thick : Inport
  h_thin : Inport  Port=2
  Compare To Constant : simulink/Logic and Bit Operations/Compare To Constant  relop=<=  const=0.01  OutDataTypeStr=boolean
  Dinamica Macchina 1 : Subsystem
  Logica Macchina 1 : Subsystem
  Switch2 : Switch  Criteria=u2 > Threshold  SaturateOnIntegerOverflow=off  InputSameDT=off
  Unit Delay : UnitDelay  HasFrameUpgradeWarning=on
  Zero : Constant  Value=0  OutDataTypeStr=Inherit: Inherit via back propagation
  l_a : Outport
  n_assi : Outport  Port=2
  h : Outport  Port=3
  Nt : Outport  Port=4
  tag scope: allarmeM1=global, statoM1=global, v1=global
  wires:
  Logica Macchina 1/3(Nt) -> Nt/1
  Logica Macchina 1/1(n_assi) -> n_assi/1
  Logica Macchina 1/2(l_a) -> l_a/1
  h_thick/1 -> Logica Macchina 1/2(h_thick)
  h_thin/1 -> Logica Macchina 1/3(h_thin)
  Logica Macchina 1/4(h) -> h/1
  [rho1] -> Dinamica Macchina 1/2(rho)
  [kc1] -> Dinamica Macchina 1/1(kc)
  Logica Macchina 1/5(Dt) -> Dinamica Macchina 1/3(Dt)
  Switch2/1 -> [allarmeM1]
  Zero/1 -> Switch2/3
  Dinamica Macchina 1/1(v2) -> Compare To Constant/1, [v1], Logica Macchina 1/1(v1)
  [cambio_lama1] -> Unit Delay/1
  Compare To Constant/1 -> Switch2/1, [statoM1]
  Unit Delay/1 -> Switch2/2

== system SCADA_Sawmill/Linea 1/Macchina 2 ==
  l_asse : Inport
  segnale_asse : Inport  Port=2
  h : Inport  Port=3
  w_asse : Inport  Port=4
  Ceil : Rounding  Operator=ceil
  Compare To Constant : simulink/Logic and Bit Operations/Compare To Constant  relop=<=  const=0.01  OutDataTypeStr=boolean
  Constant1 : Constant  Value=0
  Constant2 : Constant  Value=0
  Dinamica Macchina 2 : Subsystem
  Divide : Product  Inputs=*/
  Integrator : Integrator  ExternalReset=falling
  MATLAB Function2 : MATLAB Function  TreatAsAtomicUnit=on
  Memory : Memory
  OR : Logic  Operator=OR  IconShape=distinctive  AllPortsSameDT=off  OutDataTypeStr=boolean
  Switch : Switch  Criteria=u2 > Threshold  SaturateOnIntegerOverflow=off  InputSameDT=off
  Switch1 : Switch  Criteria=u2 > Threshold  SaturateOnIntegerOverflow=off  InputSameDT=off
  Switch2 : Switch  Criteria=u2 > Threshold  SaturateOnIntegerOverflow=off  InputSameDT=off
  Unit Delay : UnitDelay  HasFrameUpgradeWarning=on
  Zero : Constant  Value=0  OutDataTypeStr=Inherit: Inherit via back propagation
  w_asse1 : InportShadow  Port=4
  n_assi_finali : Outport
  tag scope: allarmeM2=global, larg_asse_m2_l1=global, statoM2=global, v2=global, w_cut_m2_l1=global
  wires:
  Divide/1 -> Ceil/1
  OR/1 -> Switch/2, Memory/1
  Constant2/1 -> Switch/3
  Switch/1 -> Dinamica Macchina 2/2(kc), Switch1/2
  Integrator/1 -> MATLAB Function2/1(u)
  MATLAB Function2/2(taglio) -> OR/2
  h/1 -> Dinamica Macchina 2/3(h)
  l_asse/1 -> [larg_asse_m2_l1], MATLAB Function2/3(l_asse), Dinamica Macchina 2/5(l_asse), Divide/1
  Ceil/1 -> Dinamica Macchina 2/1(n_seghe)
  Memory/1 -> Integrator/2
  [kc1] -> Switch/1
  w_asse1/1 -> [w_cut_m2_l1], Divide/2
  segnale_asse/1 -> OR/1
  w_asse/1 -> MATLAB Function2/2(w_asse)
  [rho1] -> Dinamica Macchina 2/4(rho)
  Switch1/1 -> Integrator/1
  Constant1/1 -> Switch1/3
  MATLAB Function2/1(y) -> n_assi_finali/1
  Dinamica Macchina 2/1(v2) -> Switch1/1, [v2], Compare To Constant/1
  Zero/1 -> Switch2/3
  Switch2/1 -> [allarmeM2]
  Compare To Constant/1 -> Switch2/1, [statoM2]
  [cambio_lama1] -> Unit Delay/1
  Unit Delay/1 -> Switch2/2

== system SCADA_Sawmill/Linea 1/Macchina 3 ==
  l_asse : Inport
  segnale_asse : Inport  Port=2
  h : Inport  Port=3
  w_asse : Inport  Port=4
  Ceil : Rounding  Operator=ceil
  Compare To Constant : simulink/Logic and Bit Operations/Compare To Constant  relop=<=  const=0.01  OutDataTypeStr=boolean
  Constant1 : Constant  Value=0
  Constant2 : Constant  Value=0
  Dinamica Macchina 2 : Subsystem
  Divide : Product  Inputs=*/
  Integrator : Integrator  ExternalReset=falling
  MATLAB Function2 : MATLAB Function  TreatAsAtomicUnit=on
  Memory : Memory
  OR : Logic  Operator=OR  IconShape=distinctive  AllPortsSameDT=off  OutDataTypeStr=boolean
  Switch : Switch  Criteria=u2 > Threshold  SaturateOnIntegerOverflow=off  InputSameDT=off
  Switch1 : Switch  Criteria=u2 > Threshold  SaturateOnIntegerOverflow=off  InputSameDT=off
  Switch2 : Switch  Criteria=u2 > Threshold  SaturateOnIntegerOverflow=off  InputSameDT=off
  Unit Delay : UnitDelay  HasFrameUpgradeWarning=on
  Zero : Constant  Value=0  OutDataTypeStr=Inherit: Inherit via back propagation
  w_asse1 : InportShadow  Port=4
  n_assi_finali : Outport
  tag scope: allarmeM3=global, larg_asse_m3_l1=global, statoM3=global, v3=global, w_cut_m3_l1=global
  wires:
  Divide/1 -> Ceil/1
  OR/1 -> Switch/2, Memory/1
  Constant2/1 -> Switch/3
  Switch/1 -> Dinamica Macchina 2/2(kc), Switch1/2
  Integrator/1 -> MATLAB Function2/1(u)
  MATLAB Function2/2(taglio) -> OR/2
  h/1 -> Dinamica Macchina 2/3(h)
  l_asse/1 -> [larg_asse_m3_l1], MATLAB Function2/3(l_asse), Dinamica Macchina 2/5(l_asse), Divide/1
  Ceil/1 -> Dinamica Macchina 2/1(n_seghe)
  Memory/1 -> Integrator/2
  [kc1] -> Switch/1
  w_asse1/1 -> [w_cut_m3_l1], Divide/2
  segnale_asse/1 -> OR/1
  w_asse/1 -> MATLAB Function2/2(w_asse)
  [rho1] -> Dinamica Macchina 2/4(rho)
  Switch1/1 -> Integrator/1
  Constant1/1 -> Switch1/3
  MATLAB Function2/1(y) -> n_assi_finali/1
  Compare To Constant/1 -> Switch2/1, [statoM3]
  Switch2/1 -> [allarmeM3]
  Zero/1 -> Switch2/3
  Dinamica Macchina 2/1(v2) -> Switch1/1, Compare To Constant/1, [v3]
  [cambio_lama1] -> Unit Delay/1
  Unit Delay/1 -> Switch2/2

== system SCADA_Sawmill/Linea 1/Subsystem ==
  n_assi : Inport
  h_asse : Inport  Port=2
  h_thin : Inport  Port=3
  h_thick : Inport  Port=4
  AND : Logic  IconShape=distinctive  AllPortsSameDT=off  OutDataTypeStr=boolean
  Compare To Zero : simulink/Logic and Bit Operations/Compare To Zero  relop=~=  OutDataTypeStr=boolean
  Detect Change : simulink/Logic and Bit Operations/Detect Change  vinit=0  OutDataTypeStr=boolean
  Equal : RelationalOperator  Operator===  OutDataTypeStr=boolean  RndMeth=Simplest  InputSameDT=off
  Equal1 : RelationalOperator  Operator===  OutDataTypeStr=boolean  RndMeth=Simplest  InputSameDT=off
  Scope2 : Scope
  Scope6 : Scope
  Switch{,1..3} (4 alike) : Switch  Criteria=u2 > Threshold  SaturateOnIntegerOverflow=off  InputSameDT=off
  Zero : Constant  Value=0  OutDataTypeStr=Inherit: Inherit via back propagation
  Zero1 : Constant  Value=0  OutDataTypeStr=Inherit: Inherit via back propagation
  segnale_thick : Outport
  h_thick1 : Outport  Port=2
  segnale_thin : Outport  Port=3
  h_thin1 : Outport  Port=4
  wires:
  Detect Change/1 -> Scope2/1, AND/2
  Zero/1 -> Switch/3, Switch1/3
  Switch/1 -> h_thick1/1
  n_assi/1 -> Compare To Zero/1, Detect Change/1
  Compare To Zero/1 -> AND/1
  Switch1/1 -> h_thin1/1
  Zero1/1 -> Switch2/3, Switch3/3
  h_asse/1 -> Equal1/2, Equal/2, Switch/1, Switch1/1
  Switch2/1 -> segnale_thick/1
  AND/1 -> Switch3/1, Switch2/1, Scope6/1
  Switch3/1 -> segnale_thin/1
  h_thick/1 -> Equal/1
  Equal/1 -> Switch/2, Switch2/2
  h_thin/1 -> Equal1/1
  Equal1/1 -> Switch1/2, Switch3/2

== system SCADA_Sawmill/Linea 2/Macchina 1 ==
  h_thick : Inport
  h_thin : Inport  Port=2
  Compare To Constant : simulink/Logic and Bit Operations/Compare To Constant  relop=<=  const=0.01  OutDataTypeStr=boolean
  Dinamica Macchina 1 : Subsystem
  Logica Macchina 1 : Subsystem
  Switch2 : Switch  Criteria=u2 > Threshold  SaturateOnIntegerOverflow=off  InputSameDT=off
  Unit Delay : UnitDelay  HasFrameUpgradeWarning=on
  Zero : Constant  Value=0  OutDataTypeStr=Inherit: Inherit via back propagation
  l_a : Outport
  n_assi : Outport  Port=2
  h : Outport  Port=3
  Nt : Outport  Port=4
  tag scope: allarmeM4=global, statoM4=global, v4=global
  wires:
  Logica Macchina 1/5(Dt) -> Dinamica Macchina 1/3(Dt)
  [kc2] -> Dinamica Macchina 1/1(kc)
  [rho2] -> Dinamica Macchina 1/2(rho)
  Logica Macchina 1/4(h) -> h/1
  h_thin/1 -> Logica Macchina 1/3(h_thin)
  h_thick/1 -> Logica Macchina 1/2(h_thick)
  Logica Macchina 1/2(l_a) -> l_a/1
  Logica Macchina 1/1(n_assi) -> n_assi/1
  Logica Macchina 1/3(Nt) -> Nt/1
  Dinamica Macchina 1/1(v2) -> Logica Macchina 1/1(v1), [v4], Compare To Constant/1
  [cambio_lama2] -> Unit Delay/1
  Zero/1 -> Switch2/3
  Compare To Constant/1 -> Switch2/1, [statoM4]
  Switch2/1 -> [allarmeM4]
  Unit Delay/1 -> Switch2/2

== system SCADA_Sawmill/Linea 2/Macchina 2 ==
  l_asse : Inport
  segnale_asse : Inport  Port=2
  h : Inport  Port=3
  w_asse : Inport  Port=4
  Ceil : Rounding  Operator=ceil
  Compare To Constant : simulink/Logic and Bit Operations/Compare To Constant  relop=<=  const=0.01  OutDataTypeStr=boolean
  Constant1 : Constant  Value=0
  Constant2 : Constant  Value=0
  Dinamica Macchina 2 : Subsystem
  Divide : Product  Inputs=*/
  Integrator : Integrator  ExternalReset=falling
  MATLAB Function2 : MATLAB Function  TreatAsAtomicUnit=on
  Memory : Memory
  OR : Logic  Operator=OR  IconShape=distinctive  AllPortsSameDT=off  OutDataTypeStr=boolean
  Scope : Scope
  Switch : Switch  Criteria=u2 > Threshold  SaturateOnIntegerOverflow=off  InputSameDT=off
  Switch1 : Switch  Criteria=u2 > Threshold  SaturateOnIntegerOverflow=off  InputSameDT=off
  Switch2 : Switch  Criteria=u2 > Threshold  SaturateOnIntegerOverflow=off  InputSameDT=off
  Unit Delay : UnitDelay  HasFrameUpgradeWarning=on
  Zero : Constant  Value=0  OutDataTypeStr=Inherit: Inherit via back propagation
  w_asse1 : InportShadow  Port=4
  n_assi_finali : Outport
  tag scope: allarmeM5=global, larg_asse_m2_l2=global, statoM5=global, v5=global, w_cut_m2_l2=global
  wires:
  MATLAB Function2/1(y) -> n_assi_finali/1
  Constant1/1 -> Switch1/3
  Switch1/1 -> Integrator/1
  [rho2] -> Dinamica Macchina 2/4(rho)
  w_asse/1 -> MATLAB Function2/2(w_asse)
  segnale_asse/1 -> OR/1
  w_asse1/1 -> [w_cut_m2_l2], Divide/2
  [kc2] -> Switch/1
  Memory/1 -> Integrator/2
  Ceil/1 -> Dinamica Macchina 2/1(n_seghe), Scope/1
  l_asse/1 -> Divide/1, [larg_asse_m2_l2], Dinamica Macchina 2/5(l_asse), MATLAB Function2/3(l_asse)
  h/1 -> Dinamica Macchina 2/3(h)
  MATLAB Function2/2(taglio) -> OR/2
  Integrator/1 -> MATLAB Function2/1(u)
  Switch/1 -> Switch1/2, Dinamica Macchina 2/2(kc)
  Constant2/1 -> Switch/3
  OR/1 -> Memory/1, Switch/2
  Divide/1 -> Ceil/1
  Dinamica Macchina 2/1(v2) -> Compare To Constant/1, [v5], Switch1/1
  Compare To Constant/1 -> Switch2/1, [statoM5]
  Unit Delay/1 -> Switch2/2
  Zero/1 -> Switch2/3
  Switch2/1 -> [allarmeM5]
  [cambio_lama2] -> Unit Delay/1

== system SCADA_Sawmill/Linea 2/Macchina 3 ==
  l_asse : Inport
  segnale_asse : Inport  Port=2
  h : Inport  Port=3
  w_asse : Inport  Port=4
  Ceil : Rounding  Operator=ceil
  Compare To Constant : simulink/Logic and Bit Operations/Compare To Constant  relop=<=  const=0.01  OutDataTypeStr=boolean
  Constant1 : Constant  Value=0
  Constant2 : Constant  Value=0
  Dinamica Macchina 2 : Subsystem
  Divide : Product  Inputs=*/
  Integrator : Integrator  ExternalReset=falling
  MATLAB Function2 : MATLAB Function  TreatAsAtomicUnit=on
  Memory : Memory
  OR : Logic  Operator=OR  IconShape=distinctive  AllPortsSameDT=off  OutDataTypeStr=boolean
  Switch : Switch  Criteria=u2 > Threshold  SaturateOnIntegerOverflow=off  InputSameDT=off
  Switch1 : Switch  Criteria=u2 > Threshold  SaturateOnIntegerOverflow=off  InputSameDT=off
  Switch2 : Switch  Criteria=u2 > Threshold  SaturateOnIntegerOverflow=off  InputSameDT=off
  Unit Delay : UnitDelay  HasFrameUpgradeWarning=on
  Zero : Constant  Value=0  OutDataTypeStr=Inherit: Inherit via back propagation
  w_asse1 : InportShadow  Port=4
  n_assi_finali : Outport
  tag scope: allarmeM6=global, larg_asse_m3_l2=global, statoM6=global, v6=global, w_cut_m3_l2=global
  wires:
  MATLAB Function2/1(y) -> n_assi_finali/1
  Constant1/1 -> Switch1/3
  Switch1/1 -> Integrator/1
  [rho2] -> Dinamica Macchina 2/4(rho)
  w_asse/1 -> MATLAB Function2/2(w_asse)
  segnale_asse/1 -> OR/1
  w_asse1/1 -> [w_cut_m3_l2], Divide/2
  [kc2] -> Switch/1
  Memory/1 -> Integrator/2
  Ceil/1 -> Dinamica Macchina 2/1(n_seghe)
  l_asse/1 -> Divide/1, [larg_asse_m3_l2], Dinamica Macchina 2/5(l_asse), MATLAB Function2/3(l_asse)
  h/1 -> Dinamica Macchina 2/3(h)
  MATLAB Function2/2(taglio) -> OR/2
  Integrator/1 -> MATLAB Function2/1(u)
  Switch/1 -> Switch1/2, Dinamica Macchina 2/2(kc)
  Constant2/1 -> Switch/3
  OR/1 -> Memory/1, Switch/2
  Divide/1 -> Ceil/1
  Dinamica Macchina 2/1(v2) -> Compare To Constant/1, [v6], Switch1/1
  Compare To Constant/1 -> Switch2/1, [statoM6]
  Unit Delay/1 -> Switch2/2
  Zero/1 -> Switch2/3
  Switch2/1 -> [allarmeM6]
  [cambio_lama2] -> Unit Delay/1

== system SCADA_Sawmill/Linea 2/Subsystem ==
  n_assi : Inport
  h_asse : Inport  Port=2
  h_thin : Inport  Port=3
  h_thick : Inport  Port=4
  AND : Logic  IconShape=distinctive  AllPortsSameDT=off  OutDataTypeStr=boolean
  Compare To Zero : simulink/Logic and Bit Operations/Compare To Zero  relop=~=  OutDataTypeStr=boolean
  Detect Change : simulink/Logic and Bit Operations/Detect Change  vinit=0  OutDataTypeStr=boolean
  Equal : RelationalOperator  Operator===  OutDataTypeStr=boolean  RndMeth=Simplest  InputSameDT=off
  Equal1 : RelationalOperator  Operator===  OutDataTypeStr=boolean  RndMeth=Simplest  InputSameDT=off
  Scope2 : Scope
  Scope6 : Scope
  Switch{,1..3} (4 alike) : Switch  Criteria=u2 > Threshold  SaturateOnIntegerOverflow=off  InputSameDT=off
  Zero : Constant  Value=0  OutDataTypeStr=Inherit: Inherit via back propagation
  Zero1 : Constant  Value=0  OutDataTypeStr=Inherit: Inherit via back propagation
  segnale_thick : Outport
  h_thick1 : Outport  Port=2
  segnale_thin : Outport  Port=3
  h_thin1 : Outport  Port=4
  wires:
  Equal1/1 -> Switch3/2, Switch1/2
  h_thin/1 -> Equal1/1
  Equal/1 -> Switch2/2, Switch/2
  h_thick/1 -> Equal/1
  Switch3/1 -> segnale_thin/1
  AND/1 -> Scope6/1, Switch2/1, Switch3/1
  Switch2/1 -> segnale_thick/1
  h_asse/1 -> Switch1/1, Switch/1, Equal/2, Equal1/2
  Zero1/1 -> Switch3/3, Switch2/3
  Switch1/1 -> h_thin1/1
  Compare To Zero/1 -> AND/1
  n_assi/1 -> Detect Change/1, Compare To Zero/1
  Switch/1 -> h_thick1/1
  Zero/1 -> Switch1/3, Switch/3
  Detect Change/1 -> AND/2, Scope2/1

== system SCADA_Sawmill/Linea 3/Macchina 1 ==
  h_thick : Inport
  h_thin : Inport  Port=2
  Compare To Constant : simulink/Logic and Bit Operations/Compare To Constant  relop=<=  const=0.01  OutDataTypeStr=boolean
  Dinamica Macchina 1 : Subsystem
  Logica Macchina 1 : Subsystem
  Switch2 : Switch  Criteria=u2 > Threshold  SaturateOnIntegerOverflow=off  InputSameDT=off
  Unit Delay : UnitDelay  HasFrameUpgradeWarning=on
  Zero : Constant  Value=0  OutDataTypeStr=Inherit: Inherit via back propagation
  l_a : Outport
  n_assi : Outport  Port=2
  h : Outport  Port=3
  Nt : Outport  Port=4
  tag scope: allarmeM7=global, statoM7=global, v7=global
  wires:
  Logica Macchina 1/3(Nt) -> Nt/1
  Logica Macchina 1/1(n_assi) -> n_assi/1
  Logica Macchina 1/2(l_a) -> l_a/1
  h_thick/1 -> Logica Macchina 1/2(h_thick)
  h_thin/1 -> Logica Macchina 1/3(h_thin)
  Logica Macchina 1/4(h) -> h/1
  [rho3] -> Dinamica Macchina 1/2(rho)
  [kc3] -> Dinamica Macchina 1/1(kc)
  Logica Macchina 1/5(Dt) -> Dinamica Macchina 1/3(Dt)
  [cambio_lama3] -> Unit Delay/1
  Zero/1 -> Switch2/3
  Compare To Constant/1 -> Switch2/1, [statoM7]
  Switch2/1 -> [allarmeM7]
  Dinamica Macchina 1/1(v2) -> Compare To Constant/1, [v7], Logica Macchina 1/1(v1)
  Unit Delay/1 -> Switch2/2
